simulink model "lab_2_sim_zeros"  (R2021a)
settings: Solver=VariableStepAuto  StartTime=0.0  StopTime=10.0  RelTol=1e-3
values from neighbouring files (symbols this model uses):
  B_sm = 20e3    (= 20000)    [lab_2_sm.m]
  J_sm = 600e3    (= 600000)    [lab_2_sm.m]
  K_sm = 1    [lab_2_sm.m]
settings Model: Creator=Ahmed  LastModifiedBy=Ahmed

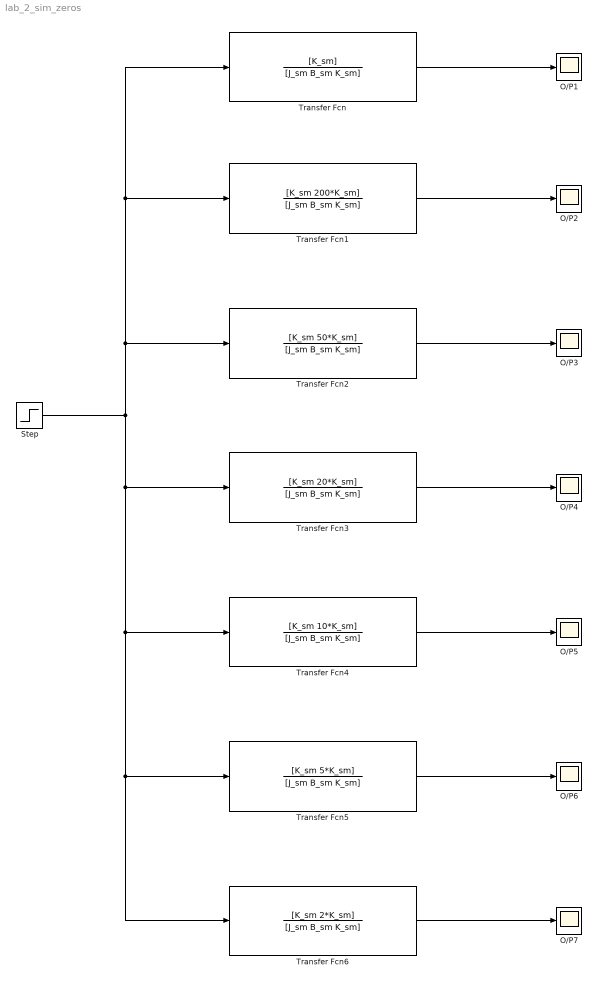
== system lab_2_sim_zeros ==
  O/P{1..7} (7 alike) : Scope
  Step : Step  Time=0  SampleTime=0
  Transfer Fcn : TransferFcn  Numerator=[K_sm]  Denominator=[J_sm B_sm K_sm]
  Transfer Fcn1 : TransferFcn  Numerator=[K_sm 200*K_sm]  Denominator=[J_sm B_sm K_sm]
  Transfer Fcn2 : TransferFcn  Numerator=[K_sm 50*K_sm]  Denominator=[J_sm B_sm K_sm]
  Transfer Fcn3 : TransferFcn  Numerator=[K_sm 20*K_sm]  Denominator=[J_sm B_sm K_sm]
  Transfer Fcn4 : TransferFcn  Numerator=[K_sm 10*K_sm]  Denominator=[J_sm B_sm K_sm]
  Transfer Fcn5 : TransferFcn  Numerator=[K_sm 5*K_sm]  Denominator=[J_sm B_sm K_sm]
  Transfer Fcn6 : TransferFcn  Numerator=[K_sm 2*K_sm]  Denominator=[J_sm B_sm K_sm]
  wires:
  Transfer Fcn3/1 -> O/P4/1
  Transfer Fcn1/1 -> O/P2/1
  Transfer Fcn/1 -> O/P1/1
  Transfer Fcn2/1 -> O/P3/1
  Transfer Fcn4/1 -> O/P5/1
  Transfer Fcn5/1 -> O/P6/1
  Transfer Fcn6/1 -> O/P7/1
  Step/1 -> Transfer Fcn2/1, Transfer Fcn1/1, Transfer Fcn/1, Transfer Fcn6/1, Transfer Fcn5/1, Transfer Fcn4/1, Transfer Fcn3/1
